simulink model "week3"  (R2020b)
settings: Solver=VariableStepAuto  StartTime=0.0  StopTime=50  RelTol=1e-3
settings Model: Creator=hp  LastModifiedBy=ASUS

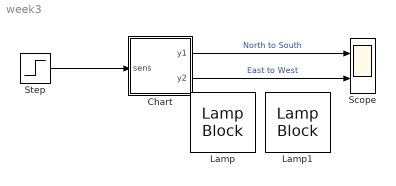
== system week3 ==
  Chart : Stateflow chart  TreatAsAtomicUnit=on
  Lamp : LampBlock
  Lamp1 : LampBlock
  Scope : Scope  NumInputPorts=2
  Step : Step  SampleTime=0
  wires:
  Chart/1(y1) -> Scope/1  "North to South"
  Chart/2(y2) -> Scope/2  "East to West"
  Step/1 -> Chart/1(sens)

== stateflow chart week3/Chart ==
  state Stop
    y1 = RED;
    y2 = GREEN;
  state StopForTraffic
    y1 = RED;
    y2 = GREEN;
  state StopToGo
    y1 = RED;
    y2 = YELLOW;
  state GoToStop
    y1 = YELLOW;
    y2 = RED;
  state Go
    y1 = GREEN;
    y2 = RED;
  (default) -> Stop
  StopForTraffic -> StopToGo : [sens]
  Stop -> StopForTraffic : after(20,tick)
  GoToStop -> Stop : after (3,tick)
  StopToGo -> Go : after(3,tick)
  Go -> GoToStop : after(10,tick)
  data: y1 output double; y2 output double; sens input double; RED constant double =1; GREEN constant double =3; YELLOW constant double =2
